simulink model "Projet_Laser"  (R2020a)
settings: Solver=VariableStepAuto  StartTime=0.0  StopTime=T-1/Fe  RelTol=1e-3
values from neighbouring files (symbols this model uses):
  F1 = 85.0059    [Projet_Laser_Game.m]    (also in Script_Signal_Carre.m = 85000)
  F2 = 90    [Projet_Laser_Game.m]
  F3 = 94.9868    [Projet_Laser_Game.m]
  F4 = 100    [Projet_Laser_Game.m]
  F5 = 115.0159    [Projet_Laser_Game.m]
  F6 = 120    [Projet_Laser_Game.m]
  Fe = 320    [Projet_Laser_Game.m]    (also in ScriptDFT.m = 128; Script_Signal_Carre.m = 320000)
settings Model: Creator=rmoulin  LastModifiedBy=rmoulin

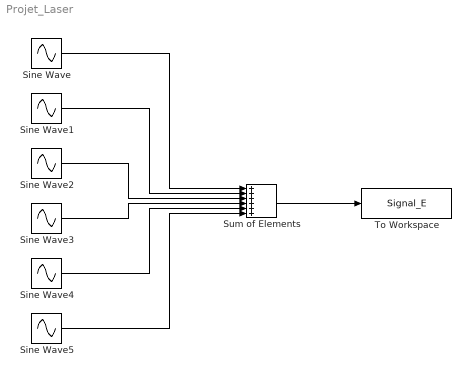
== system Projet_Laser ==
  Sine Wave : Sin  Frequency=2*pi*F1  SampleTime=0
  Sine Wave1 : Sin  Frequency=2*pi*F2  SampleTime=0
  Sine Wave2 : Sin  Frequency=2*pi*F3  SampleTime=0
  Sine Wave3 : Sin  Frequency=2*pi*F4  SampleTime=0
  Sine Wave4 : Sin  Frequency=2*pi*F5  SampleTime=0
  Sine Wave5 : Sin  Frequency=2*pi*F6  SampleTime=0
  Sum of Elements : Sum  Inputs=++++++
  To Workspace : ToWorkspace  VariableName=Signal_E  SaveFormat=Timeseries  SampleTime=1/Fe
  wires:
  Sine Wave/1 -> Sum of Elements/1
  Sine Wave1/1 -> Sum of Elements/2
  Sine Wave2/1 -> Sum of Elements/3
  Sine Wave3/1 -> Sum of Elements/4
  Sine Wave4/1 -> Sum of Elements/5
  Sine Wave5/1 -> Sum of Elements/6
  Sum of Elements/1 -> To Workspace/1
